simulink model "Sim_Particle_Controller_first_order"  (R2017b)
settings: Solver=VariableStepAuto  StartTime=0.0  StopTime=10.0  RelTol=1e-3
settings Model: Creator=nilst  LastModifiedBy=nilst

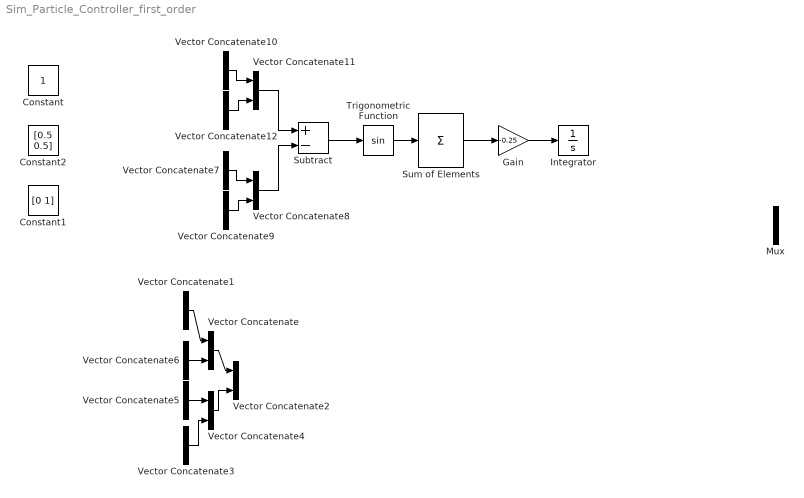
== system Sim_Particle_Controller_first_order ==
  Constant : Constant
  Constant1 : Constant  Value=[0 1]
  Constant2 : Constant  Value=[0.5 0.5]
  Gain : Gain  Gain=-0.25
  Integrator : Integrator
  Mux : Mux
  Subtract : Sum  Inputs=+-
  Sum of Elements : Sum  Inputs=+
  Trigonometric Function : Trigonometry
  Vector Concatenate{,1..12} (13 alike) : Concatenate
  wires:
  Gain/1 -> Integrator/1
  Sum of Elements/1 -> Gain/1
  Trigonometric Function/1 -> Sum of Elements/1
  Subtract/1 -> Trigonometric Function/1
  Vector Concatenate1/1 -> Vector Concatenate/1
  Vector Concatenate6/1 -> Vector Concatenate/2
  Vector Concatenate5/1 -> Vector Concatenate4/1
  Vector Concatenate3/1 -> Vector Concatenate4/2
  Vector Concatenate/1 -> Vector Concatenate2/1
  Vector Concatenate4/1 -> Vector Concatenate2/2
  Vector Concatenate7/1 -> Vector Concatenate8/1
  Vector Concatenate9/1 -> Vector Concatenate8/2
  Vector Concatenate8/1 -> Subtract/2
  Vector Concatenate10/1 -> Vector Concatenate11/1
  Vector Concatenate12/1 -> Vector Concatenate11/2
  Vector Concatenate11/1 -> Subtract/1
